simulink model "cap3ex3_11"  (R2017b)
settings: Solver=VariableStepAuto  StartTime=0.0  StopTime=10.0  RelTol=1e-3
settings Model: Creator=rafael  LastModifiedBy=rafael

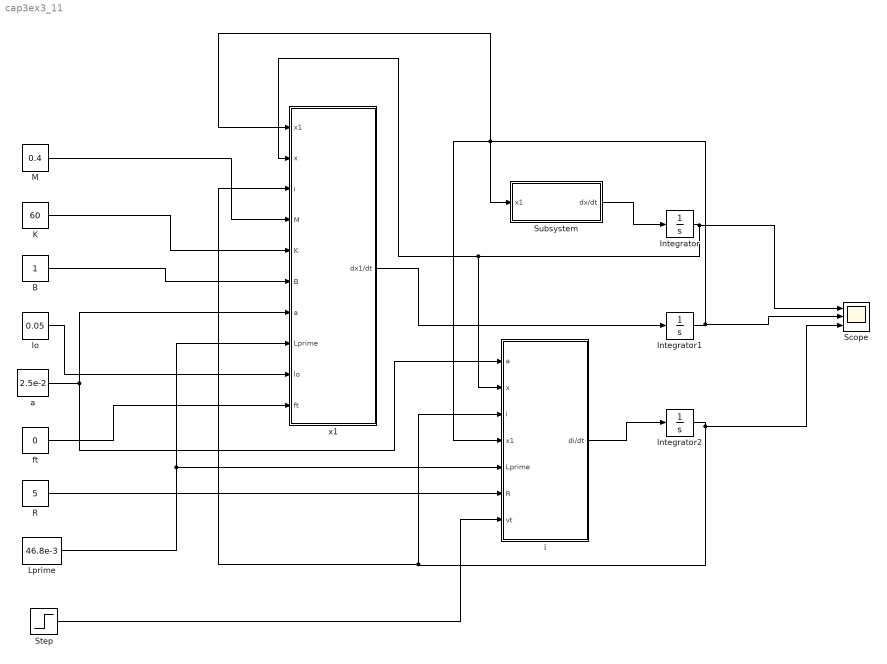
== system cap3ex3_11 ==
  B : Constant
  Integrator : Integrator  InitialCondition=0.1
  Integrator1 : Integrator
  Integrator2 : Integrator
  K : Constant  Value=60
  Lprime : Constant  Value=46.8e-3
  M : Constant  Value=0.4
  R : Constant  Value=5
  Scope : Scope  NumInputPorts=3
  Step : Step  SampleTime=0
  Subsystem : Subsystem
  a : Constant  Value=2.5e-2
  ft : Constant  Value=0
  i : Subsystem
  lo : Constant  Value=0.05
  x1 : Subsystem
  wires:
  Lprime/1 -> i/5(Lprime), x1/8(Lprime)
  R/1 -> i/6(R)
  ft/1 -> x1/10(ft)
  a/1 -> x1/7(a), i/1(a)
  B/1 -> x1/6(B)
  K/1 -> x1/5(K)
  M/1 -> x1/4(M)
  x1/1(dx1/dt) -> Integrator1/1
  Integrator1/1 -> Scope/2, i/4(x1), Subsystem/1(x1), x1/1(x1)
  i/1(di/dt) -> Integrator2/1
  Integrator2/1 -> Scope/3, x1/3(i), i/3(i)
  Subsystem/1(dx/dt) -> Integrator/1
  Integrator/1 -> Scope/1, x1/2(x), i/2(x)
  Step/1 -> i/7(vt)
  lo/1 -> x1/9(lo)

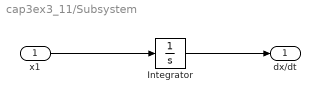
== system cap3ex3_11/Subsystem ==
  x1 : Inport
  Integrator : Integrator
  dx/dt : Outport
  wires:
  x1/1 -> Integrator/1
  Integrator/1 -> dx/dt/1

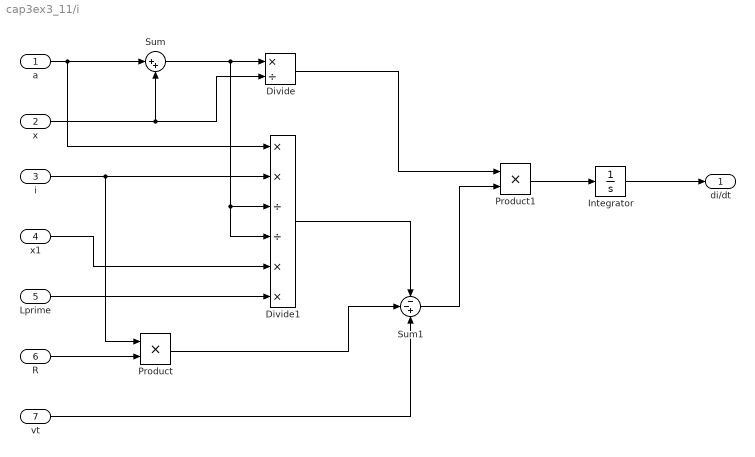
== system cap3ex3_11/i ==
  a : Inport
  x : Inport  Port=2
  i : Inport  Port=3
  x1 : Inport  Port=4
  Lprime : Inport  Port=5
  R : Inport  Port=6
  vt : Inport  Port=7
  Divide : Product  Inputs=*/
  Divide1 : Product  Inputs=**//**
  Integrator : Integrator
  Product : Product
  Product1 : Product
  Sum : Sum  Inputs=|++
  Sum1 : Sum  Inputs=--+
  di/dt : Outport
  wires:
  a/1 -> Divide1/1, Sum/1
  x/1 -> Divide/2, Sum/2
  Sum/1 -> Divide1/4, Divide1/3, Divide/1
  i/1 -> Product/1, Divide1/2
  x1/1 -> Divide1/5
  Lprime/1 -> Divide1/6
  R/1 -> Product/2
  Divide1/1 -> Sum1/1
  Product/1 -> Sum1/2
  vt/1 -> Sum1/3
  Sum1/1 -> Product1/2
  Divide/1 -> Product1/1
  Integrator/1 -> di/dt/1
  Product1/1 -> Integrator/1

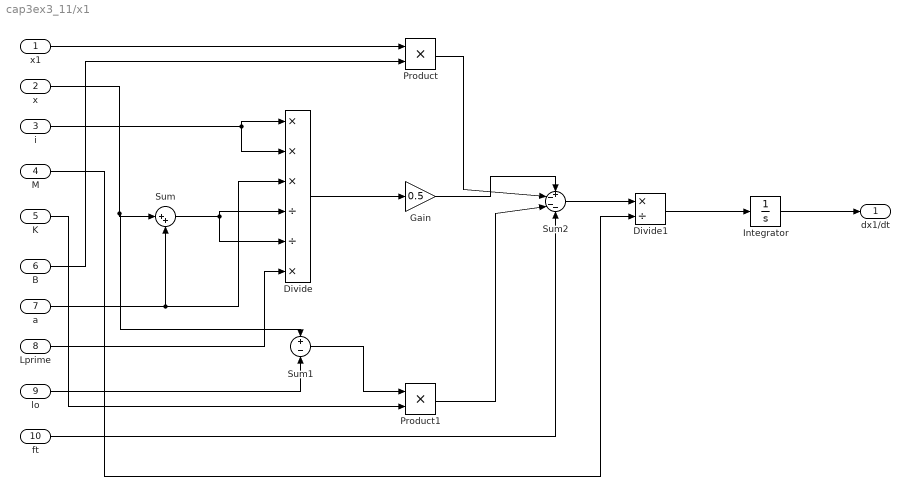
== system cap3ex3_11/x1 ==
  x1 : Inport
  x : Inport  Port=2
  i : Inport  Port=3
  M : Inport  Port=4
  K : Inport  Port=5
  B : Inport  Port=6
  a : Inport  Port=7
  Lprime : Inport  Port=8
  lo : Inport  Port=9
  ft : Inport  Port=10
  Divide : Product  Inputs=***//*
  Divide1 : Product  Inputs=*/
  Gain : Gain  Gain=0.5
  Integrator : Integrator
  Product : Product
  Product1 : Product
  Sum : Sum  Inputs=|++
  Sum1 : Sum  Inputs=+-
  Sum2 : Sum  Inputs=+---
  dx1/dt : Outport
  wires:
  i/1 -> Divide/1, Divide/2
  x/1 -> Sum1/1, Sum/1
  a/1 -> Divide/3, Sum/2
  Sum/1 -> Divide/4, Divide/5
  Lprime/1 -> Divide/6
  Divide/1 -> Gain/1
  B/1 -> Product/2
  x1/1 -> Product/1
  lo/1 -> Sum1/2
  K/1 -> Product1/2
  Sum1/1 -> Product1/1
  Gain/1 -> Sum2/1
  Product/1 -> Sum2/2
  Product1/1 -> Sum2/3
  ft/1 -> Sum2/4
  Sum2/1 -> Divide1/1
  M/1 -> Divide1/2
  Divide1/1 -> Integrator/1
  Integrator/1 -> dx1/dt/1
